simulink model "exercise_1_alternativo"  (R2023a)
settings: Solver=VariableStepAuto  StartTime=0.0  StopTime=T0  RelTol=1e-3
InitFcn:
  | %% Initial conditions
  | % Cubesat 3U x=0.1 m; y=0.1 m; z=0.3 m; m=0.7+0.7+0.7=2.25 kg
  | x = 0.1;
  | y = 0.1;
  | z = 0.3;
  | m = 2.25;
  | 
  | % Calculation of moments of inertia Ix, Iy, Iz
  | Iz = m/12 * (x^2+y^2);   % kg*m^2
  | Ix = m/12 * (z^2+y^2);   % kg*m^2
  | Iy = Ix;                 % kg*m^2
  | 
  | I=[Ix 0 0 ; 0 Iy 0; 0 0 Iz]; % inertia matrix
  | 
  | % Orbital radius r0=700 km and calculation of orbital period
  | % T=2pi*sqrt(r^3/mu) s
  | re = 6371;   % km
  | r0 = re+700; % km
  | mu = 398600; % km^3/s^2
  | 
  | % Orbital period
  | T0 = 2*pi*sqrt(r0^3/mu); % s
  | 
  | % Sinusoidal torques Tx=5e-8 * cos(t), Ty=2e-8 * sin(t), Tz=3e-8 * sin(2t)
  | Ax = 5e-8;
  | omegax = 1e-2;
  | phasex = pi/2;
  | 
  | Ay = 2e-8;
  | omegay = 1e-2;
  | phasey = pi/2;
  | 
  | Az = 3e-8;
  | omegaz = 1e-2;
  | phasez = pi/2;
  | 
  | % Nadir pointing quaternion
  | qIC=[0;0;0;1];
  | 
  | % Orbital velocity initial
  | omega_oi = 2*pi/T0;
  | omega_bi_IC = [0;-omega_oi;0];
libraries: matrix_library x1, aerolibutil x1
settings Model: Creator=modeand16864  LastModifiedBy=comun
settings DebuggingCC: UnderspecifiedInitializationDetection=Classic  MergeDetectMultiDrivingBlocksExec=none
settings ModelReferenceCC: PropagateSignalLabelsOutOfModel=off

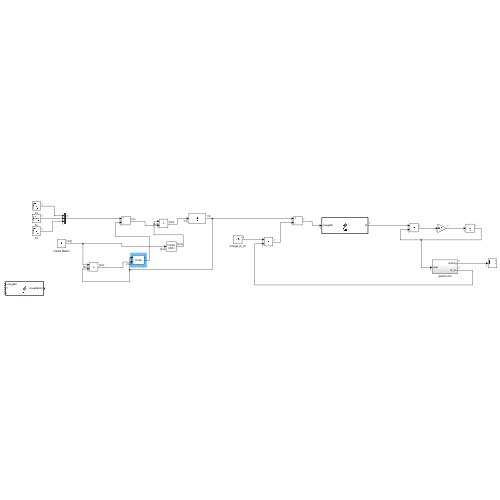
[thumbnail: Simulink's stored preview of the top-level diagram]
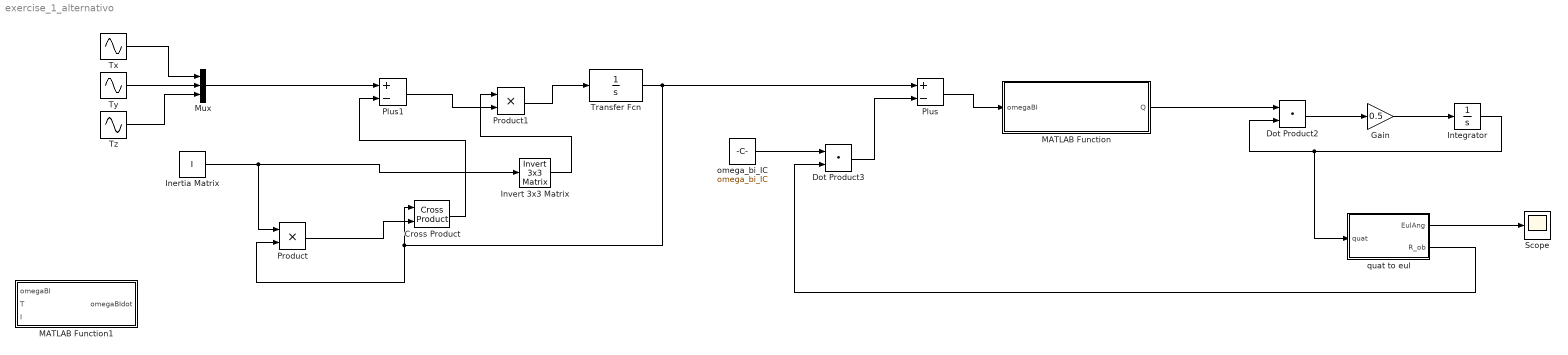
== system exercise_1_alternativo ==
  Cross Product : matrix_library/Cross Product
  Dot Product2 : DotProduct  OutDataTypeStr=Inherit: Inherit via internal rule
  Dot Product3 : DotProduct  OutDataTypeStr=Inherit: Inherit via internal rule
  Gain : Gain  Gain=0.5
  Inertia Matrix : Constant  Value=I
  Integrator : Integrator
  Invert 3x3 Matrix : aerolibutil/Invert  3x3 Matrix
  MATLAB Function : MATLAB Function  TreatAsAtomicUnit=on
  MATLAB Function1 : MATLAB Function  TreatAsAtomicUnit=on
  Mux : Mux  Inputs=3
  Plus : Sum  Inputs=+-
  Plus1 : Sum  Inputs=+-
  Product : Product
  Product1 : Product
  Scope : Scope
  Transfer Fcn : TransferFcn  Denominator=[1 0]
  Tx : Sin  Amplitude=Ax  Frequency=omegax  Phase=phasex  SampleTime=0
  Ty : Sin  Amplitude=Ay  Frequency=omegay  Phase=phasey  SampleTime=0
  Tz : Sin  Amplitude=Az  Frequency=omegaz  Phase=phasez  SampleTime=0
  omega_bi_IC : Constant  Value=omega_bi_IC
  quat to eul : Subsystem
  wires:
  MATLAB Function/1(Q) -> Dot Product2/1
  Gain/1 -> Integrator/1
  Dot Product3/1 -> Plus/2
  Plus/1 -> MATLAB Function/1(omegaBI)
  Dot Product2/1 -> Gain/1
  quat to eul/1(EulAng) -> Scope/1
  quat to eul/2(R_ob) -> Dot Product3/2
  Integrator/1 -> Dot Product2/2, quat to eul/1(quat)
  Transfer Fcn/1 -> Product/2, Cross Product/1, Plus/1
  omega_bi_IC/1 -> Dot Product3/1
  Inertia Matrix/1 -> Product/1, Invert 3x3 Matrix/1
  Tx/1 -> Mux/1
  Ty/1 -> Mux/2
  Tz/1 -> Mux/3
  Mux/1 -> Plus1/1
  Product/1 -> Cross Product/2
  Cross Product/1 -> Plus1/2
  Product1/1 -> Transfer Fcn/1
  Plus1/1 -> Product1/2
  Invert 3x3 Matrix/1 -> Product1/1

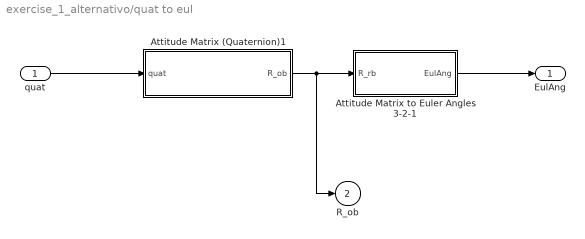
== system exercise_1_alternativo/quat to eul ==
  quat : Inport
  Attitude Matrix (Quaternion)1 : Subsystem
  Attitude Matrix to Euler Angles 3-2-1 : Subsystem
  EulAng : Outport  VectorParamsAs1DForOutWhenUnconnected=off
  R_ob : Outport  Port=2
  wires:
  Attitude Matrix to Euler Angles 3-2-1/1(EulAng) -> EulAng/1
  Attitude Matrix (Quaternion)1/1(R_ob) -> Attitude Matrix to Euler Angles 3-2-1/1(R_rb), R_ob/1
  quat/1 -> Attitude Matrix (Quaternion)1/1(quat)

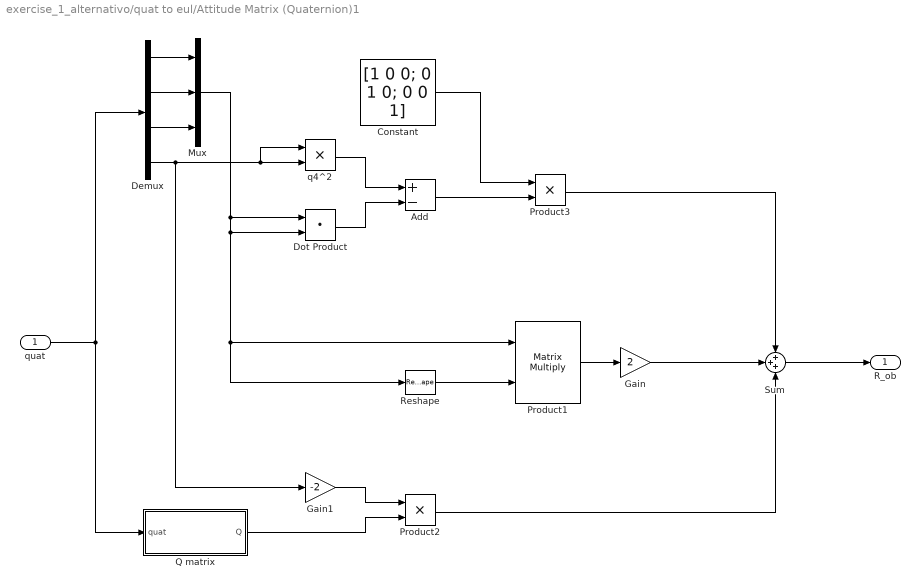
== system exercise_1_alternativo/quat to eul/Attitude Matrix (Quaternion)1 ==
  quat : Inport
  Add : Sum  Inputs=+-
  Constant : Constant  Value=[1 0 0; 0 1 0; 0 0 1]
  Demux : Demux
  Dot Product : DotProduct  OutDataTypeStr=Inherit: Inherit via internal rule
  Gain : Gain  Gain=2
  Gain1 : Gain  Gain=-2
  Mux : Mux  Inputs=3
  Product1 : Product  Multiplication=Matrix(*)  RndMeth=Zero
  Product2 : Product  RndMeth=Zero
  Product3 : Product  RndMeth=Zero
  Q matrix : Subsystem
  Reshape : Reshape  OutputDimensionality=Row vector (2-D)
  Sum : Sum  Inputs=+++
  q4^2 : Product  RndMeth=Zero
  R_ob : Outport  VectorParamsAs1DForOutWhenUnconnected=off
  wires:
  quat/1 -> Demux/1, Q matrix/1(quat)
  Demux/4 -> q4^2/2, q4^2/1, Gain1/1
  Reshape/1 -> Product1/2
  Product1/1 -> Gain/1
  Gain/1 -> Sum/2
  q4^2/1 -> Add/1
  Dot Product/1 -> Add/2
  Product2/1 -> Sum/3
  Add/1 -> Product3/2
  Sum/1 -> R_ob/1
  Constant/1 -> Product3/1
  Product3/1 -> Sum/1
  Demux/1 -> Mux/1
  Demux/2 -> Mux/2
  Demux/3 -> Mux/3
  Mux/1 -> Dot Product/1, Reshape/1, Product1/1, Dot Product/2
  Gain1/1 -> Product2/1
  Q matrix/1(Q) -> Product2/2

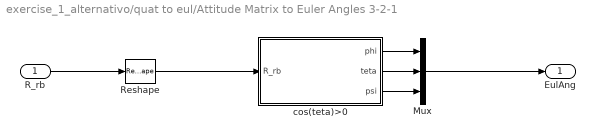
== system exercise_1_alternativo/quat to eul/Attitude Matrix to Euler Angles 3-2-1 ==
  R_rb : Inport
  Mux : Mux  Inputs=3
  Reshape : Reshape  OutputDimensionality=Column vector (2-D)
  cos(teta)>0 : Subsystem
  EulAng : Outport  VectorParamsAs1DForOutWhenUnconnected=off
  wires:
  cos(teta)>0/2(teta) -> Mux/2
  cos(teta)>0/1(phi) -> Mux/1
  cos(teta)>0/3(psi) -> Mux/3
  Mux/1 -> EulAng/1
  Reshape/1 -> cos(teta)>0/1(R_rb)
  R_rb/1 -> Reshape/1

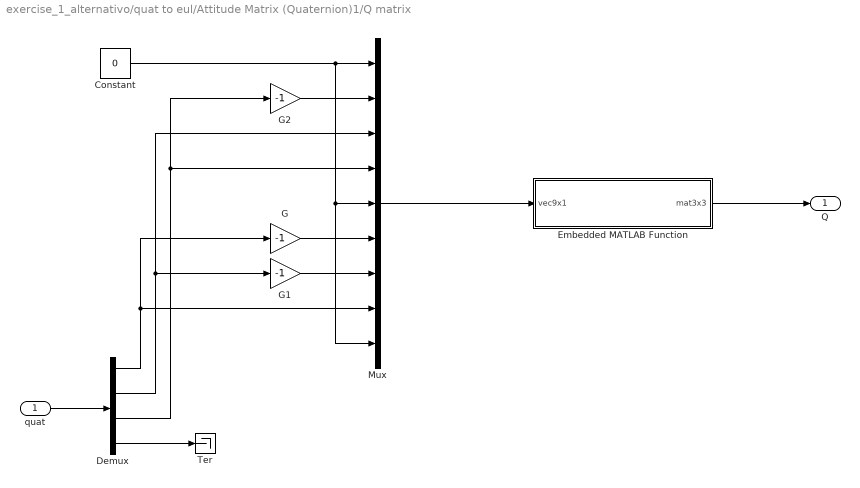
== system exercise_1_alternativo/quat to eul/Attitude Matrix (Quaternion)1/Q matrix ==
  quat : Inport
  Constant : Constant  Value=0
  Demux : Demux
  Embedded MATLAB Function : MATLAB Function  TreatAsAtomicUnit=on
  G : Gain  Gain=-1
  G1 : Gain  Gain=-1
  G2 : Gain  Gain=-1
  Mux : Mux  Inputs=9
  Ter : Terminator
  Q : Outport  VectorParamsAs1DForOutWhenUnconnected=off
  wires:
  Demux/4 -> Ter/1
  quat/1 -> Demux/1
  Constant/1 -> Mux/9, Mux/5, Mux/1
  Demux/1 -> G/1, Mux/8
  G1/1 -> Mux/7
  Demux/2 -> G1/1, Mux/3
  G/1 -> Mux/6
  G2/1 -> Mux/2
  Demux/3 -> G2/1, Mux/4
  Embedded MATLAB Function/1(mat3x3) -> Q/1
  Mux/1 -> Embedded MATLAB Function/1(vec9x1)

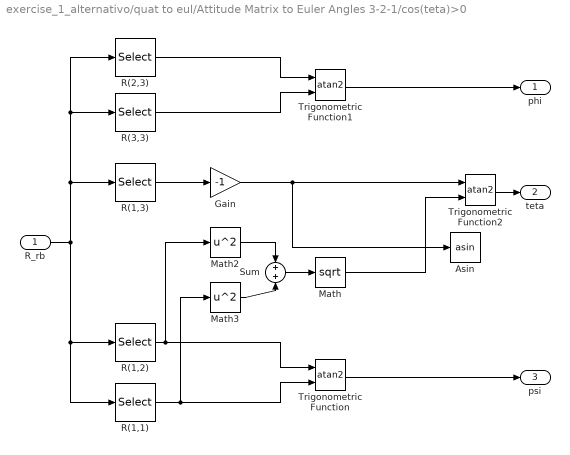
== system exercise_1_alternativo/quat to eul/Attitude Matrix to Euler Angles 3-2-1/cos(teta)>0 ==
  R_rb : Inport
  Asin : Trigonometry  Operator=asin
  Gain : Gain  Gain=-1
  Math : Math  Operator=sqrt  SignedPower=on
  Math2 : Math  Operator=square  SignedPower=on
  Math3 : Math  Operator=square  SignedPower=on
  R(1,1) : Selector  InputPortWidth=9  IndexOptions=Index vector (dialog)  Indices=[1]  OutputSizes=1
  R(1,2) : Selector  InputPortWidth=9  IndexOptions=Index vector (dialog)  Indices=[4]  OutputSizes=1
  R(1,3) : Selector  InputPortWidth=9  IndexOptions=Index vector (dialog)  Indices=[7]  OutputSizes=1
  R(2,3) : Selector  InputPortWidth=9  IndexOptions=Index vector (dialog)  Indices=[8]  OutputSizes=1
  R(3,3) : Selector  InputPortWidth=9  IndexOptions=Index vector (dialog)  Indices=[9]  OutputSizes=1
  Sum : Sum
  Trigonometric Function : Trigonometry  Operator=atan2
  Trigonometric Function1 : Trigonometry  Operator=atan2
  Trigonometric Function2 : Trigonometry  Operator=atan2
  phi : Outport  VectorParamsAs1DForOutWhenUnconnected=off
  teta : Outport  Port=2  VectorParamsAs1DForOutWhenUnconnected=off
  psi : Outport  Port=3  VectorParamsAs1DForOutWhenUnconnected=off
  wires:
  R_rb/1 -> R(1,1)/1, R(1,2)/1, R(1,3)/1, R(3,3)/1, R(2,3)/1
  R(1,2)/1 -> Trigonometric Function/1, Math2/1
  R(1,1)/1 -> Trigonometric Function/2, Math3/1
  R(2,3)/1 -> Trigonometric Function1/1
  R(3,3)/1 -> Trigonometric Function1/2
  R(1,3)/1 -> Gain/1
  Gain/1 -> Asin/1, Trigonometric Function2/1
  Math2/1 -> Sum/1
  Math3/1 -> Sum/2
  Sum/1 -> Math/1
  Math/1 -> Trigonometric Function2/2
  Trigonometric Function1/1 -> phi/1
  Trigonometric Function2/1 -> teta/1
  Trigonometric Function/1 -> psi/1

== matlab function exercise_1_alternativo/MATLAB Function ==
  data: omegaBI input; Q output
function Q = fcn(omegaBI)

Wbox = omegaBI(1);
Wboy = omegaBI(2);
Wboz = omegaBI(3);

Q=[0 Wboz -Wboy Wbox; -Wboz 0 Wbox Wboy; Wboy -Wbox 0 Wboz; -Wbox -Wboy -Wboz 0];

== matlab function exercise_1_alternativo/MATLAB Function1 ==
  data: omegaBI input; T input; I input; omegaBIdot output
function omegaBIdot = fcn(omegaBI, T, I)


omegaBIdot = I'*(T-cross(omegaBI, I*omegaBI));

== matlab function exercise_1_alternativo/quat to eul/Attitude Matrix (Quaternion)1/Q matrix/Embedded MATLAB Function ==
  data: vec9x1 input; mat3x3 output
function mat3x3 = vec2mat(vec9x1)
%#eml

s = size(vec9x1);

if s(1)>s(2)
    vec = vec9x1';
else
    vec = vec9x1;
end

mat3x3 = [vec(1:3); vec(4:6); vec(7:9)];
